simulink model "VehicleSteering_sim_PolePlacement"  (R2017b)
settings: Solver=VariableStepAuto  StartTime=0.0  StopTime=10.0  RelTol=1e-3
undefined symbols (not defined in the file): A, B, C, D, K, kr
settings Model: Creator=jofr  LastModifiedBy=jofr

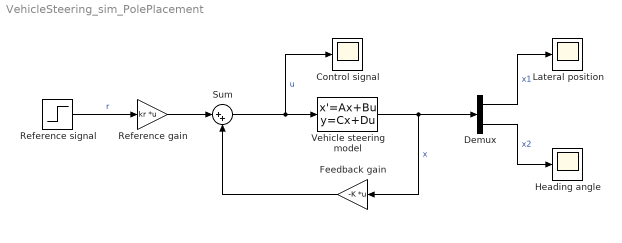
== system VehicleSteering_sim_PolePlacement ==
  Control signal : Scope
  Demux : Demux  Outputs=2
  Feedback gain : Gain  Gain=-K  Multiplication=Matrix(K*u)
  Heading angle : Scope
  Lateral position : Scope
  Reference gain : Gain  Gain=kr  Multiplication=Matrix(K*u)
  "Reference signal " : Step  SampleTime=0
  Sum : Sum  Inputs=|++
  Vehicle steering model : StateSpace  A=A  B=B  C=C  D=D  InitialCondition=0
  wires:
  Vehicle steering model/1 -> Demux/1, Feedback gain/1  "x"
  Sum/1 -> Control signal/1, Vehicle steering model/1  "u"
  Feedback gain/1 -> Sum/2
  Reference gain/1 -> Sum/1
  Demux/1 -> Lateral position/1  "x1"
  Demux/2 -> Heading angle/1  "x2"
  "Reference signal "/1 -> Reference gain/1  "r"
